simulink model "makeOcB_th"  (R2020a)
settings: Solver=VariableStepAuto  StartTime=0.0  StopTime=0  RelTol=1e-3
libraries: makeOcB_cl x1
settings Model: Creator=Ayaz  LastModifiedBy=Ayaz

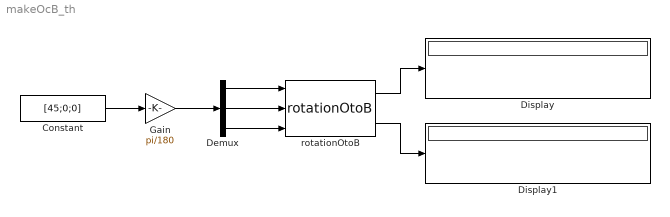
== system makeOcB_th ==
  Constant : Constant  Value=[45;0;0]
  Demux : Demux  Outputs=3
  Display : Display
  Display1 : Display
  Gain : Gain  Gain=pi/180
  rotationOtoB : makeOcB_cl/rotationOtoB  SystemSampleTime=-1  Latency=0  AutoFrameSizeCalculation=off
  wires:
  Demux/1 -> rotationOtoB/1
  Demux/2 -> rotationOtoB/2
  Demux/3 -> rotationOtoB/3
  Constant/1 -> Gain/1
  Gain/1 -> Demux/1
  rotationOtoB/1 -> Display/1
  rotationOtoB/2 -> Display1/1
